simulink model "raibert_hopper_2d"  (R2014b)
settings: Solver=FixedStepDiscrete  StartTime=0.0  StopTime=inf  FixedStep=sample_time  RelTol=1e-3
undefined symbols (not defined in the file): boom_mount_angle, boom_pelvis_offset_angle, contact_threshold, control_start_time, d_y_boom_com_offset, desired_torso_angle, dt_thrust, dx_avg_desired, dx_avg_samples, dx_desired_step, extra_leg_damping, F_thrust, fcut_contact, g, h_boom, HIP_MTR_MAX_CONT_TORQUE, initial_dt, k_placement, k_sea, kd_flight, kd_lateral, kd_leg_angle, kd_leg_length_secondary, kd_torso, kd_virtual, kp_flight_max, kp_flight_min, kp_lateral, kp_leg_angle, kp_leg_length_secondary, kp_torso, kp_virtual, l0_virtual, l_boom_projected, l_max, l_min, l_retract, l_seg, l_yaw_center_to_pelvis, lambda1, lambda2, lateral_offset, lateral_target_angle_left, lateral_target_angle_right, leg_length_secondary, loaded_threshold, m_leg_motor, m_total_real, max_leg_angle, max_torque_lateral, max_torque_sagittal, maximum_lateral_angle, min_leg_angle, minimum_lateral_angle, sample_time, t_flight, x_limit
libraries: simulink x7
(part 1 of 2)
settings Model: xpc_rtwmakecfg_data=_xpcethercatlib_  BufferReuse=off  Creator=wmartin  LastModifiedBy=wmartin
settings SolverCC: EnableConcurrentExecution=on
settings DataIOCC: MaxDataPoints=1000000000  SaveFormat=StructureWithTime
settings OptimizationCC: BlockReduction=off  OptimizeBlockIOStorage=off  BufferReuse=off  GlobalBufferReuse=off  ExpressionFolding=off  ExpressionDepthLimit=2147483647  LocalBlockOutputs=off  SimCompilerOptimization=On
settings DebuggingCC: UnderspecifiedInitializationDetection=Classic  MergeDetectMultiDrivingBlocksExec=none  StateNameClashWarn=warning
settings HardwareCC: ProdIntDivRoundTo=Zero  ProdEndianess=LittleEndian  ProdLongLongMode=on  ProdHWDeviceType=Generic->32-bit x86 compatible
settings ModelReferenceCC: UpdateModelReferenceTargets=IfOutOfDate  EnableParallelModelReferenceBuilds=on
settings RTWCC: SystemTargetFile=slrt.tlc  TemplateMakefile=slrt_default_tmf  Description=Simulink Real-Time  RTWVerbose=off  ProcessScript=slrt_make_rtw_hook  RTWCompilerOptimization=On
settings CodeAppCC: MaxIdLength=256
settings SimulinkRealTimeCC: GeneratePreprocessorConditionals=Disable all  EnableShiftOperators=on  RL32LogBufSizeModifier=100000000

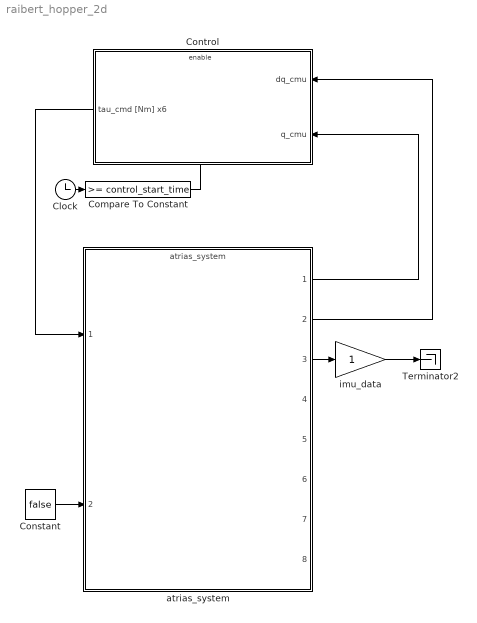
== system raibert_hopper_2d ==
  Clock : Clock
  Compare To Constant : simulink/Logic and Bit Operations/Compare To Constant  relop=>=  const=control_start_time  OutDataTypeStr=boolean
  Constant : Constant  Value=false
  Control : Subsystem
  Terminator2 : Terminator
  atrias_system : ModelReference  ModelNameDialog=atrias_system  SimulationMode=Normal  ModelReferenceVersion=1.2644  CopyOfModelName=atrias_system  DefaultDataLogging=on
  imu_data : Gain
  wires:
  Clock/1 -> Compare To Constant/1
  Compare To Constant/1 -> Control/Enable
  atrias_system/1 -> Control/2(q_cmu)
  atrias_system/2 -> Control/1(dq_cmu)
  Constant/1 -> atrias_system/2
  Control/1(tau_cmd [Nm] x6) -> atrias_system/1
  imu_data/1 -> Terminator2/1
  atrias_system/3 -> imu_data/1

== system raibert_hopper_2d/Control ==
  dq_cmu : Inport
  q_cmu : Inport  Port=2
  Enable : EnablePort  StatesWhenEnabling=reset
  Actuator Control : ModelReference  ModelNameDialog=actuator_control  SimulationMode=Normal  ModelReferenceVersion=1.25  CopyOfModelName=actuator_control  DefaultDataLogging=on
  Behavior Control : Subsystem
  Constant : Constant  Value=[true true true true]  OutDataTypeStr=boolean
  tau_cmd [Nm] x6 : Outport  InitialOutput=[0 0 0 0 0 0]
  wires:
  q_cmu/1 -> Behavior Control/2(q_cmu), Actuator Control/3
  dq_cmu/1 -> Behavior Control/1(dq_cmu), Actuator Control/4
  Behavior Control/1(motor_torque_cmd) -> Actuator Control/1
  Actuator Control/1 -> tau_cmd [Nm] x6/1
  Constant/1 -> Actuator Control/2

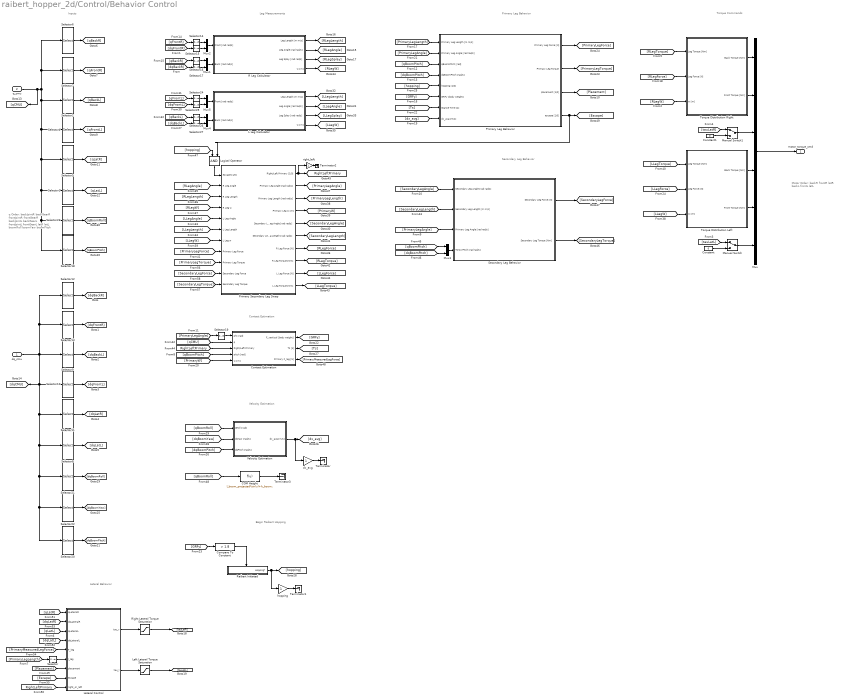
== system raibert_hopper_2d/Control/Behavior Control ==
  note: Begin Raibert Hopping
  note: Velocity Estimation
  note: Contact Estimation
  note: Leg Measurements
  note: Lateral Behavior
  note: Torque Commands
  note: Secondary Leg Behavior
  note: Primary Leg Behavior
  note: Inputs
  note: q Order:
      |
      | backJointR
      | backGearR
      | frontJointR
      | frontGearR
      |
      | backJointL
      | backGearL
      | frontJointL
      | frontGearL
      |
      | latR
      | latL
      |
      | boomRoll
      | boomYaw
      | boomPitch
  note: Motor Order:
      |
      | backR
      | frontR
      | latR
      | backL
      | frontL
      | latL
  dq_cmu : Inport
  q_cmu : Inport  Port=2
  COM Height : Fcn  Expr=l_boom_projected*sin(u)+h_boom;
  Compare To Constant : simulink/Logic and Bit Operations/Compare To Constant  relop=>  const=1.8  OutDataTypeStr=boolean
  Constant : Constant  Value=0
  Constant1 : Constant  Value=0
  Contact Estimation : Subsystem
  L Leg Calculator : Subsystem
  Lateral Control : MATLAB Function  TreatAsAtomicUnit=on
  Left Lateral Torque Saturation : Saturate  UpperLimit=max_torque_lateral  LowerLimit=-max_torque_lateral
      settings: AttributesFormatString=Top: %<UpperLimit>\nBottom: %<LowerLimit>
  Logical Operator : Logic  IconShape=distinctive  AllPortsSameDT=off  OutDataTypeStr=boolean
  Manual Switch : ManualSwitch
  Manual Switch1 : ManualSwitch
  Mux : Mux  Inputs=6
  Mux{1..5} (5 alike) : Mux  Inputs=2
  Primary Leg Behavior : Subsystem
  Primary Secondary Leg Swap : Subsystem
  R Leg Calculator : Subsystem
  Raibert Initiated : Subsystem
  Right Lateral Torque Saturation : Saturate  UpperLimit=max_torque_lateral  LowerLimit=-max_torque_lateral
      settings: AttributesFormatString=Top: %<UpperLimit>\nBottom: %<LowerLimit>
  Secondary Leg Behavior : Subsystem
  Selector{,14..17,19,24..27} (10 alike) : Selector  InputPortWidth=2  Indices=[1]
  Selector1 : Selector  InputPortWidth=13  Indices=[10]
  Selector10 : Selector  InputPortWidth=13  Indices=[7 8]
  Selector11 : Selector  InputPortWidth=13  Indices=[9]
  Selector12 : Selector  InputPortWidth=13  Indices=[1 2]
  Selector13 : Selector  InputPortWidth=13  Indices=[3 4]
  Selector18 : Selector  InputPortWidth=13  Indices=[13]
  Selector2 : Selector  InputPortWidth=13  Indices=[5 6]
  Selector20 : Selector  InputPortWidth=13  Indices=[13]
  Selector21 : Selector  InputPortWidth=13  Indices=[11]
  Selector22 : Selector  InputPortWidth=13  Indices=[12]
  Selector23 : Selector  InputPortWidth=13  Indices=[11]
  Selector4 : Selector  InputPortWidth=13  Indices=[7 8]
  Selector5 : Selector  InputPortWidth=13  Indices=[9]
  Selector6 : Selector  InputPortWidth=13  Indices=[1 2]
  Selector7 : Selector  InputPortWidth=13  Indices=[3 4]
  Selector8 : Selector  InputPortWidth=13  Indices=[10]
  Selector9 : Selector  InputPortWidth=13  Indices=[5 6]
  Terminator{,1..3} (4 alike) : Terminator
  Torque Distribution Left : Subsystem
  Torque Distribution Right : Subsystem
  Velocity Estimation : Subsystem
  dx_avg : Gain
  hopping : Gain
  right_left : Gain
  motor_torque_cmd : Outport  OutputWhenDisabled=reset  InitialOutput=[0 0 0 0 0 0]
  tag scope: RightLeftPrimary=global
  wires:
  Compare To Constant/1 -> Raibert Initiated/Enable
  COM Height/1 -> Terminator3/1
  [qBoomRoll] -> COM Height/1
  Logical Operator/1 -> Primary Secondary Leg Swap/1(escape [1/0])
  [hopping] -> Logical Operator/1
  right_left/1 -> Terminator2/1
  Mux3/1 -> Secondary Leg Behavior/4(Torso Pitch [rad rad/s])
  [dqBoomPitch] -> Mux3/2
  [qBoomPitch] -> Mux3/1
  [SecondaryLegLength] -> Secondary Leg Behavior/2(Secondary Leg Length [m m/s])
  [SecondaryLegAngle] -> Secondary Leg Behavior/1(Secondary Leg Angle [rad rad/s])
  [PrimaryLegAngle] -> Secondary Leg Behavior/3(Primary Leg Angle [rad rad/s])
  Secondary Leg Behavior/2(Secondary Leg Torque [Nm]) -> [SecondaryLegTorque]
  Secondary Leg Behavior/1(Secondary Leg Force [N]) -> [SecondaryLegForce]
  [RightLeftPrimary] -> Contact Estimation/3(Right/Left Primary)
  [qCMU] -> Contact Estimation/2(q)
  [LLegW] -> Torque Distribution Left/3(w [m])
  [LLegForce] -> Torque Distribution Left/2(Leg Force [N])
  [LLegTorque] -> Torque Distribution Left/1(Leg Torque [Nm])
  Torque Distribution Left/2(Front Torque [Nm]) -> Mux/5
  Torque Distribution Left/1(Back Torque [Nm]) -> Mux/4
  hopping/1 -> Terminator1/1
  dx_avg/1 -> Terminator/1
  [dqBoomPitch] -> Velocity Estimation/3(dqPitch [rad/s])
  [dqBoomYaw] -> Velocity Estimation/2(dqYaw [rad/s])
  [qBoomRoll] -> Velocity Estimation/1(qRoll [rad])
  Velocity Estimation/1(dx_avg [m/s]) -> [dx_avg], dx_avg/1
  Primary Leg Behavior/2(Primary Leg Torque) -> [PrimaryLegTorque]
  Primary Leg Behavior/1(Primary Leg Force [N]) -> [PrimaryLegForce]
  [dx_avg] -> Primary Leg Behavior/8(dx_avg [m/s])
  [Ts] -> Primary Leg Behavior/7(Stance Time [s])
  [PrimaryLegAngle] -> Primary Leg Behavior/2(Primary Leg Angle [rad rad/s])
  [dqBoomPitch] -> Primary Leg Behavior/4(dqBoomPitch [rad/s])
  [qBoomPitch] -> Primary Leg Behavior/3(qBoomPitch [rad])
  [GRFy] -> Primary Leg Behavior/6(GRFy [body weight])
  [hopping] -> Primary Leg Behavior/5(hopping [1/0])
  [PrimaryLegLength] -> Primary Leg Behavior/1(Primary Leg Length [m m/s])
  Primary Secondary Leg Swap/1(Right/Left Primary [1/0]) -> [RightLeftPrimary], right_left/1
  Primary Leg Behavior/4(escape [1/0]) -> [Escape], Logical Operator/2
  Primary Secondary Leg Swap/10(L Leg Torque [Nm]) -> [LLegTorque]
  Primary Secondary Leg Swap/9(L Leg Force [N]) -> [LLegForce]
  Primary Secondary Leg Swap/8(R Leg Torque [Nm]) -> [RLegTorque]
  Primary Secondary Leg Swap/7(R Leg Force [N]) -> [RLegForce]
  Primary Secondary Leg Swap/4(Primary Leg w [m]) -> [PrimaryW]
  Primary Secondary Leg Swap/3(Primary Leg Length [rad rad/s]) -> [PrimaryLegLength]
  Primary Secondary Leg Swap/2(Primary Leg Angle [rad rad/s]) -> [PrimaryLegAngle]
  Primary Secondary Leg Swap/6(Secondary Leg Length [rad rad/s]) -> [SecondaryLegLength]
  Primary Secondary Leg Swap/5(Secondary Leg Angle [rad rad/s]) -> [SecondaryLegAngle]
  [SecondaryLegTorque] -> Primary Secondary Leg Swap/11(Secondary Leg Torque)
  [SecondaryLegForce] -> Primary Secondary Leg Swap/10(Secondary Leg Force)
  [PrimaryLegTorque] -> Primary Secondary Leg Swap/9(Primary Leg Torque)
  [PrimaryLegForce] -> Primary Secondary Leg Swap/8(Primary Leg Force)
  [RLegW] -> Primary Secondary Leg Swap/4(R Leg w)
  [RLegLength] -> Primary Secondary Leg Swap/3(R Leg Length)
  [RLegAngle] -> Primary Secondary Leg Swap/2(R Leg Angle)
  [LLegW] -> Primary Secondary Leg Swap/7(L Leg w)
  [LLegLength] -> Primary Secondary Leg Swap/6(L Leg Length)
  [LLegAngle] -> Primary Secondary Leg Swap/5(L Leg Angle)
  L Leg Calculator/4(w [m]) -> [LLegW]
  R Leg Calculator/4(w [m]) -> [RLegW]
  Selector26/1 -> Mux4/1
  Selector27/1 -> Mux4/2
  Selector25/1 -> Mux5/2
  Selector24/1 -> Mux5/1
  L Leg Calculator/3(Leg Splay [rad rad/s]) -> [LLegSplay]
  L Leg Calculator/2(Leg Angle [rad rad/s]) -> [LLegAngle]
  L Leg Calculator/1("Leg Length [m m/s] ") -> [LLegLength]
  Mux4/1 -> L Leg Calculator/2(Back [rad rad/s])
  Mux5/1 -> L Leg Calculator/1(Front [rad rad/s])
  [dqFrontL] -> Selector25/1
  [qFrontL] -> Selector24/1
  [dqBackL] -> Selector27/1
  [qBackL] -> Selector26/1
  Selector23/1 -> [qBoomRoll]
  Selector21/1 -> [dqBoomRoll]
  dq_cmu/1 -> Selector9/1, Selector13/1, Selector12/1, [dqCMU], Selector10/1, Selector11/1, Selector8/1, Selector21/1, Selector22/1, Selector20/1
  Raibert Initiated/1(Hopping?) -> [hopping], hopping/1
  [GRFy] -> Compare To Constant/1
  Contact Estimation/2(Ts [s]) -> [Ts]
  Selector22/1 -> [dqBoomYaw]
  [RLegTorque] -> Torque Distribution Right/1(Leg Torque [Nm])
  [RLegForce] -> Torque Distribution Right/2(Leg Force [N])
  Selector20/1 -> [dqBoomPitch]
  Contact Estimation/1(F_vertical [body weight]) -> [GRFy]
  Selector19/1 -> Contact Estimation/1(phi [rad])
  [PrimaryLegAngle] -> Selector19/1
  [qBoomPitch] -> Contact Estimation/4(pitch [rad])
  Selector18/1 -> [qBoomPitch]
  q_cmu/1 -> [qCMU], Selector1/1, Selector23/1, Selector18/1, Selector5/1, Selector4/1, Selector2/1, Selector7/1, Selector6/1
  [PrimaryW] -> Contact Estimation/5(w [m])
  Selector16/1 -> Mux1/1
  Selector17/1 -> Mux1/2
  Selector15/1 -> Mux2/2
  Selector14/1 -> Mux2/1
  [RLegW] -> Torque Distribution Right/3(w [m])
  [tauLatL] -> Manual Switch/1
  [tauLatR] -> Manual Switch1/1
  Torque Distribution Right/2(Front Torque [Nm]) -> Mux/2
  Torque Distribution Right/1(Back Torque [Nm]) -> Mux/1
  R Leg Calculator/3(Leg Splay [rad rad/s]) -> [RLegSplay]
  R Leg Calculator/2(Leg Angle [rad rad/s]) -> [RLegAngle]
  R Leg Calculator/1("Leg Length [m m/s] ") -> [RLegLength]
  Mux1/1 -> R Leg Calculator/2(Back [rad rad/s])
  Mux2/1 -> R Leg Calculator/1(Front [rad rad/s])
  [dqFrontR] -> Selector15/1
  [qFrontR] -> Selector14/1
  [dqBackR] -> Selector17/1
  [qBackR] -> Selector16/1
  Selector10/1 -> [dqFrontL]
  Selector9/1 -> [dqBackL]
  Selector13/1 -> [dqFrontR]
  Selector12/1 -> [dqBackR]
  Selector11/1 -> [dqLatR]
  Selector8/1 -> [dqLatL]
  Mux/1 -> motor_torque_cmd/1
  Manual Switch1/1 -> Mux/3
  Manual Switch/1 -> Mux/6
  Constant/1 -> Manual Switch/2
  Constant1/1 -> Manual Switch1/2
  Selector5/1 -> [qLatR]
  Selector1/1 -> [qLatL]
  Selector6/1 -> [qBackR]
  Selector7/1 -> [qFrontR]
  Selector2/1 -> [qBackL]
  Selector4/1 -> [qFrontL]
  Primary Leg Behavior/3(placement [1/0]) -> [Placement]
  Lateral Control/1(tau_r) -> Right Lateral Torque Saturation/1
  Lateral Control/2(tau_l) -> Left Lateral Torque Saturation/1
  [Placement] -> Lateral Control/7(placement)
  [RightLeftPrimary] -> Lateral Control/9(right_or_left)
  [qLatR] -> Lateral Control/1(qLateralR)
  [qLatL] -> Lateral Control/3(qLateralL)
  [dqLatL] -> Lateral Control/4(dqLateralL)
  [dqLatR] -> Lateral Control/2(dqLateralR)
  [PrimaryLegLength] -> Selector/1
  [PrimaryMeasuredLegForce] -> Lateral Control/5(F_leg)
  Right Lateral Torque Saturation/1 -> [tauLatR]
  Left Lateral Torque Saturation/1 -> [tauLatL]
  Contact Estimation/3(Primary F_leg [N]) -> [PrimaryMeasuredLegForce]
  Selector/1 -> Lateral Control/6(l_leg)
  [Escape] -> Lateral Control/8(escape)

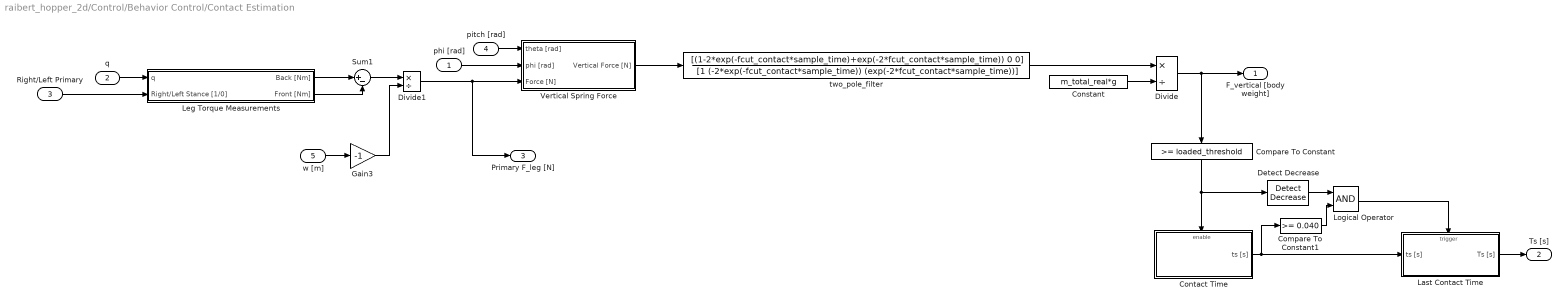
== system raibert_hopper_2d/Control/Behavior Control/Contact Estimation ==
  phi [rad] : Inport
  q : Inport  Port=2
  Right/Left Primary : Inport  Port=3
  pitch [rad] : Inport  Port=4
  w [m] : Inport  Port=5
  Compare To Constant : simulink/Logic and Bit Operations/Compare To Constant  relop=>=  const=loaded_threshold  OutDataTypeStr=boolean
  Compare To Constant1 : simulink/Logic and Bit Operations/Compare To Constant  relop=>=  const=0.040  OutDataTypeStr=boolean
  Constant : Constant  Value=m_total_real*g
  Contact Time : Subsystem
  Detect Decrease : simulink/Logic and Bit Operations/Detect Decrease  vinit=0.0  InputProcessing=Inherited  OutDataTypeStr=boolean
  Divide : Product  Inputs=*/
  Divide1 : Product  Inputs=*/
  Gain3 : Gain  Gain=-1
  Last Contact Time : Subsystem
  Leg Torque Measurements : Subsystem
  Logical Operator : Logic  AllPortsSameDT=off  OutDataTypeStr=boolean
  Sum1 : Sum  Inputs=|+-
  Vertical Spring Force : Subsystem
  two_pole_filter : DiscreteTransferFcn  Numerator=[(1-2*exp(-fcut_contact*sample_time)+exp(-2*fcut_contact*sample_time)) 0 0]  Denominator=[1 (-2*exp(-fcut_contact*sample_time)) (exp(-2*fcut_contact*sample_time))]  SampleTime=sample_time
  F_vertical [body weight] : Outport
  Ts [s] : Outport  Port=2
  Primary F_leg [N] : Outport  Port=3
  wires:
  Right/Left Primary/1 -> Leg Torque Measurements/2(Right/Left Stance [1/0])
  Compare To Constant1/1 -> Logical Operator/2
  Detect Decrease/1 -> Logical Operator/1
  Logical Operator/1 -> Last Contact Time/Trigger
  Divide/1 -> Compare To Constant/1, F_vertical [body weight]/1
  Compare To Constant/1 -> Contact Time/Enable, Detect Decrease/1
  Contact Time/1(ts [s]) -> Compare To Constant1/1, Last Contact Time/1(ts [s])
  Last Contact Time/1(Ts [s]) -> Ts [s]/1
  phi [rad]/1 -> Vertical Spring Force/2(phi [rad])
  Gain3/1 -> Divide1/2
  w [m]/1 -> Gain3/1
  pitch [rad]/1 -> Vertical Spring Force/1(theta [rad])
  Divide1/1 -> Primary F_leg [N]/1, Vertical Spring Force/3(Force [N])
  Sum1/1 -> Divide1/1
  Leg Torque Measurements/2(Front [Nm]) -> Sum1/2
  Leg Torque Measurements/1(Back [Nm]) -> Sum1/1
  q/1 -> Leg Torque Measurements/1(q)
  two_pole_filter/1 -> Divide/1
  Constant/1 -> Divide/2
  Vertical Spring Force/1(Vertical Force [N]) -> two_pole_filter/1

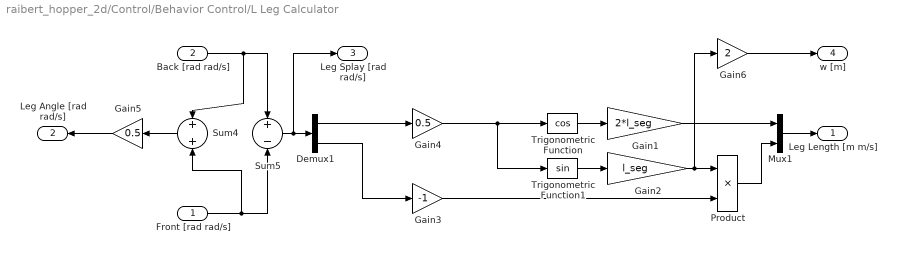
== system raibert_hopper_2d/Control/Behavior Control/L Leg Calculator ==
  Front [rad rad/s] : Inport
  Back [rad rad/s] : Inport  Port=2
  Demux1 : Demux  Outputs=2
  Gain1 : Gain  Gain=2*l_seg
  Gain2 : Gain  Gain=l_seg
  Gain3 : Gain  Gain=-1
  Gain4 : Gain  Gain=0.5
  Gain5 : Gain  Gain=0.5
  Gain6 : Gain  Gain=2
  Mux1 : Mux  Inputs=2
  Product : Product  RndMeth=Zero
  Sum4 : Sum  Inputs=+|+
  Sum5 : Sum  Inputs=+|-
  Trigonometric Function : Trigonometry  Operator=cos
  Trigonometric Function1 : Trigonometry
  "Leg Length [m m/s] " : Outport
  Leg Angle [rad rad/s] : Outport  Port=2
  Leg Splay [rad rad/s] : Outport  Port=3
  w [m] : Outport  Port=4
  wires:
  Gain6/1 -> w [m]/1
  Gain4/1 -> Trigonometric Function1/1, Trigonometric Function/1
  Trigonometric Function/1 -> Gain1/1
  Gain1/1 -> Mux1/1
  Trigonometric Function1/1 -> Gain2/1
  Product/1 -> Mux1/2
  Front [rad rad/s]/1 -> Sum5/2, Sum4/2
  Back [rad rad/s]/1 -> Sum4/1, Sum5/1
  Demux1/2 -> Gain3/1
  Gain3/1 -> Product/2
  Demux1/1 -> Gain4/1
  Gain2/1 -> Product/1, Gain6/1
  Sum5/1 -> Leg Splay [rad rad/s]/1, Demux1/1
  Mux1/1 -> "Leg Length [m m/s] "/1
  Sum4/1 -> Gain5/1
  Gain5/1 -> Leg Angle [rad rad/s]/1

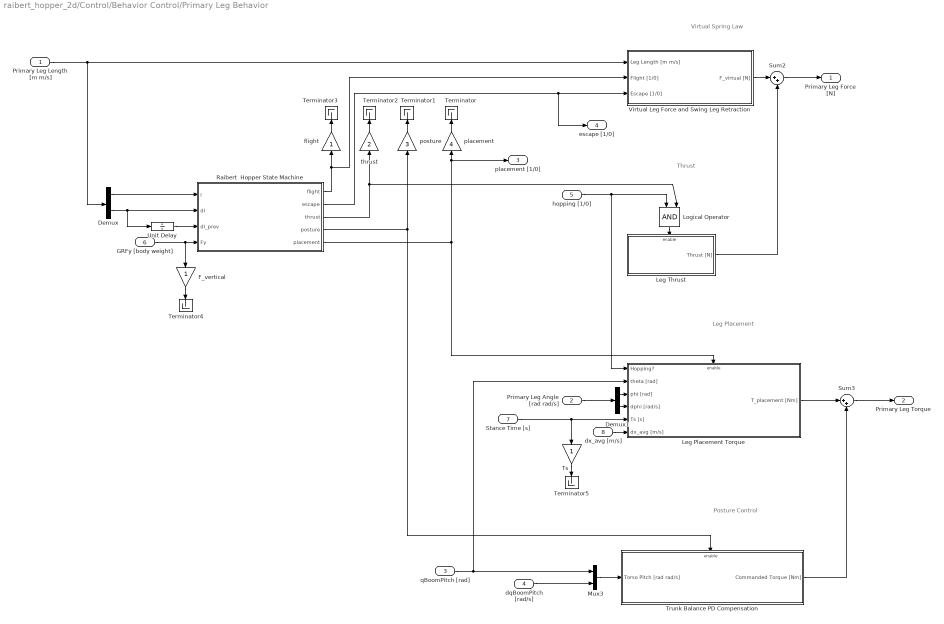
== system raibert_hopper_2d/Control/Behavior Control/Primary Leg Behavior ==
  note: Leg Placement
  note: Posture Control
  note: Thrust
  note: Virtual Spring Law
  Primary Leg Length [m m/s] : Inport
  Primary Leg Angle [rad rad/s] : Inport  Port=2
  qBoomPitch [rad] : Inport  Port=3
  dqBoomPitch [rad/s] : Inport  Port=4
  hopping [1/0] : Inport  Port=5
  GRFy [body weight] : Inport  Port=6
  Stance Time [s] : Inport  Port=7
  dx_avg [m/s] : Inport  Port=8
  Demux : Demux  Outputs=2
  Demux1 : Demux  Outputs=2
  F_vertical : Gain
  Leg Placement Torque : Subsystem
  Leg Thrust : Subsystem
  Logical Operator : Logic  IconShape=distinctive  AllPortsSameDT=off  OutDataTypeStr=boolean
  Mux3 : Mux  Inputs=2
  Raibert  Hopper State Machine : State Transition Table  TreatAsAtomicUnit=on
  Sum2 : Sum  Inputs=|++
  Sum3 : Sum  Inputs=|++
  Terminator{,1..5} (6 alike) : Terminator
  Trunk Balance PD Compensation : Subsystem
  Ts : Gain
  Unit Delay : UnitDelay  SampleTime=-1
  Virtual Leg Force and Swing Leg Retraction : Subsystem
  flight : Gain
  placement : Gain  Gain=4
  posture : Gain  Gain=3
  thrust : Gain  Gain=2
  Primary Leg Force [N] : Outport
  Primary Leg Torque : Outport  Port=2
  placement [1/0] : Outport  Port=3  OutDataTypeStr=boolean
  escape [1/0] : Outport  Port=4
  wires:
  hopping [1/0]/1 -> Logical Operator/1, Leg Placement Torque/1(Hopping?)
  Ts/1 -> Terminator5/1
  Demux/1 -> Raibert  Hopper State Machine/1(l)
  flight/1 -> Terminator3/1
  F_vertical/1 -> Terminator4/1
  Primary Leg Length [m m/s]/1 -> Virtual Leg Force and Swing Leg Retraction/1(Leg Length [m m/s]), Demux/1
  thrust/1 -> Terminator2/1
  posture/1 -> Terminator1/1
  Logical Operator/1 -> Leg Thrust/Enable
  Raibert  Hopper State Machine/5(placement) -> placement [1/0]/1, placement/1, Leg Placement Torque/Enable
  Stance Time [s]/1 -> Ts/1, Leg Placement Torque/5(Ts [s])
  Primary Leg Angle [rad rad/s]/1 -> Demux1/1
  Demux1/2 -> Leg Placement Torque/4(dphi [rad/s])
  Demux1/1 -> Leg Placement Torque/3(phi [rad])
  dx_avg [m/s]/1 -> Leg Placement Torque/6(dx_avg [m/s])
  Sum3/1 -> Primary Leg Torque/1
  Leg Placement Torque/1(T_placement [Nm]) -> Sum3/1
  Raibert  Hopper State Machine/2(escape) -> Virtual Leg Force and Swing Leg Retraction/3(Escape [1/0]), escape [1/0]/1
  Virtual Leg Force and Swing Leg Retraction/1(F_virtual [N]) -> Sum2/1
  Raibert  Hopper State Machine/1(flight) -> Virtual Leg Force and Swing Leg Retraction/2(Flight [1/0]), flight/1
  Sum2/1 -> Primary Leg Force [N]/1
  Leg Thrust/1(Thrust [N]) -> Sum2/2
  Raibert  Hopper State Machine/3(thrust) -> thrust/1, Logical Operator/2
  Demux/2 -> Raibert  Hopper State Machine/2(dl), Unit Delay/1
  GRFy [body weight]/1 -> Raibert  Hopper State Machine/4(Fy), F_vertical/1
  Unit Delay/1 -> Raibert  Hopper State Machine/3(dl_prev)
  Trunk Balance PD Compensation/1(Commanded Torque [Nm]) -> Sum3/2
  dqBoomPitch [rad/s]/1 -> Mux3/2
  qBoomPitch [rad]/1 -> Leg Placement Torque/2(theta [rad]), Mux3/1
  Mux3/1 -> Trunk Balance PD Compensation/1(Torso Pitch [rad rad/s])
  Raibert  Hopper State Machine/4(posture) -> posture/1, Trunk Balance PD Compensation/Enable
  placement/1 -> Terminator/1

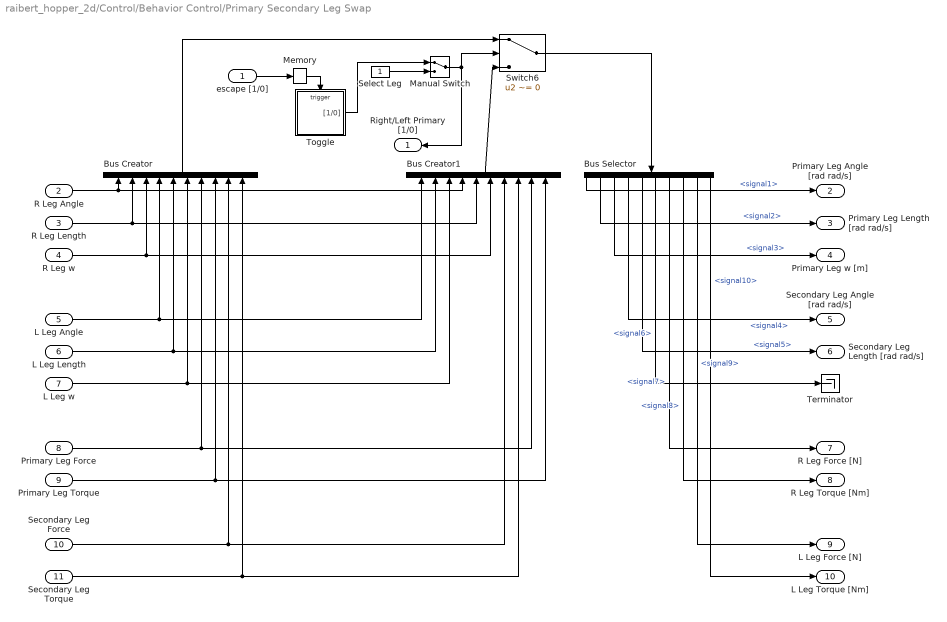
== system raibert_hopper_2d/Control/Behavior Control/Primary Secondary Leg Swap ==
  escape [1/0] : Inport
  R Leg Angle : Inport  Port=2
  R Leg Length : Inport  Port=3
  R Leg w : Inport  Port=4
  L Leg Angle : Inport  Port=5
  L Leg Length : Inport  Port=6
  L Leg w : Inport  Port=7
  Primary Leg Force : Inport  Port=8
  Primary Leg Torque : Inport  Port=9
  Secondary Leg Force : Inport  Port=10
  Secondary Leg Torque : Inport  Port=11
  Bus Creator : BusCreator  Inputs=10
  Bus Creator1 : BusCreator  Inputs=10
  Bus Selector : BusSelector  OutputSignals=signal1,signal2,signal3,signal4,signal5,signal6,signal7,signal8,signal9,signal10
  Manual Switch : ManualSwitch
  Memory : Memory  InheritSampleTime=on
  Select Leg : Constant  OutDataTypeStr=boolean
  Switch6 : Switch  Criteria=u2 ~= 0  ZeroCross=off
  Terminator : Terminator
  Toggle : Subsystem
  Right/Left Primary [1/0] : Outport
  Primary Leg Angle [rad rad/s] : Outport  Port=2
  Primary Leg Length [rad rad/s] : Outport  Port=3
  Primary Leg w [m] : Outport  Port=4
  Secondary Leg Angle [rad rad/s] : Outport  Port=5
  Secondary Leg Length [rad rad/s] : Outport  Port=6
  R Leg Force [N] : Outport  Port=7
  R Leg Torque [Nm] : Outport  Port=8
  L Leg Force [N] : Outport  Port=9
  L Leg Torque [Nm] : Outport  Port=10
  wires:
  Memory/1 -> Toggle/Trigger
  Toggle/1("[1/0]") -> Manual Switch/1
  Manual Switch/1 -> Right/Left Primary [1/0]/1, Switch6/2
  Select Leg/1 -> Manual Switch/2
  Bus Selector/10 -> L Leg Torque [Nm]/1  "<signal10>"
  Bus Selector/9 -> L Leg Force [N]/1  "<signal9>"
  Bus Selector/8 -> R Leg Torque [Nm]/1  "<signal8>"
  Bus Selector/7 -> R Leg Force [N]/1  "<signal7>"
  Bus Selector/6 -> Terminator/1  "<signal6>"
  Bus Selector/5 -> Secondary Leg Length [rad rad/s]/1  "<signal5>"
  Bus Selector/4 -> Secondary Leg Angle [rad rad/s]/1  "<signal4>"
  Bus Selector/3 -> Primary Leg w [m]/1  "<signal3>"
  Bus Selector/2 -> Primary Leg Length [rad rad/s]/1  "<signal2>"
  Bus Selector/1 -> Primary Leg Angle [rad rad/s]/1  "<signal1>"
  L Leg Angle/1 -> Bus Creator1/1, Bus Creator/4
  L Leg Length/1 -> Bus Creator1/2, Bus Creator/5
  Primary Leg Force/1 -> Bus Creator/7, Bus Creator1/9
  R Leg w/1 -> Bus Creator/3, Bus Creator1/6
  R Leg Angle/1 -> Bus Creator/1, Bus Creator1/4
  L Leg w/1 -> Bus Creator1/3, Bus Creator/6
  R Leg Length/1 -> Bus Creator/2, Bus Creator1/5
  escape [1/0]/1 -> Memory/1
  Secondary Leg Force/1 -> Bus Creator/9, Bus Creator1/7
  Secondary Leg Torque/1 -> Bus Creator/10, Bus Creator1/8
  Primary Leg Torque/1 -> Bus Creator/8, Bus Creator1/10
  Bus Creator/1 -> Switch6/1
  Bus Creator1/1 -> Switch6/3
  Switch6/1 -> Bus Selector/1

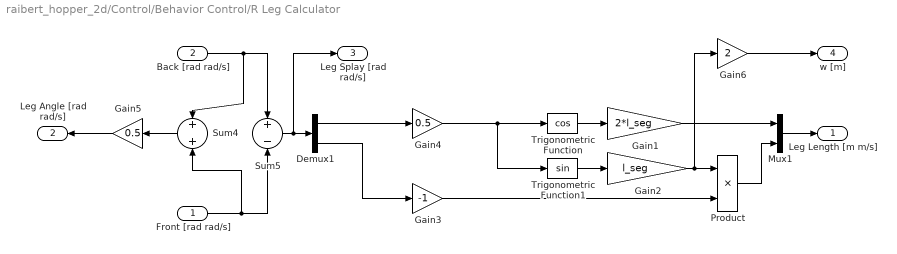
== system raibert_hopper_2d/Control/Behavior Control/R Leg Calculator ==
  Front [rad rad/s] : Inport
  Back [rad rad/s] : Inport  Port=2
  Demux1 : Demux  Outputs=2
  Gain1 : Gain  Gain=2*l_seg
  Gain2 : Gain  Gain=l_seg
  Gain3 : Gain  Gain=-1
  Gain4 : Gain  Gain=0.5
  Gain5 : Gain  Gain=0.5
  Gain6 : Gain  Gain=2
  Mux1 : Mux  Inputs=2
  Product : Product  RndMeth=Zero
  Sum4 : Sum  Inputs=+|+
  Sum5 : Sum  Inputs=+|-
  Trigonometric Function : Trigonometry  Operator=cos
  Trigonometric Function1 : Trigonometry
  "Leg Length [m m/s] " : Outport
  Leg Angle [rad rad/s] : Outport  Port=2
  Leg Splay [rad rad/s] : Outport  Port=3
  w [m] : Outport  Port=4
  wires:
  Gain5/1 -> Leg Angle [rad rad/s]/1
  Sum4/1 -> Gain5/1
  Mux1/1 -> "Leg Length [m m/s] "/1
  Sum5/1 -> Demux1/1, Leg Splay [rad rad/s]/1
  Gain2/1 -> Gain6/1, Product/1
  Demux1/1 -> Gain4/1
  Gain3/1 -> Product/2
  Demux1/2 -> Gain3/1
  Back [rad rad/s]/1 -> Sum5/1, Sum4/1
  Front [rad rad/s]/1 -> Sum4/2, Sum5/2
  Product/1 -> Mux1/2
  Trigonometric Function1/1 -> Gain2/1
  Gain1/1 -> Mux1/1
  Trigonometric Function/1 -> Gain1/1
  Gain4/1 -> Trigonometric Function/1, Trigonometric Function1/1
  Gain6/1 -> w [m]/1

== system raibert_hopper_2d/Control/Behavior Control/Raibert Initiated ==
  Enable : EnablePort  StatesWhenEnabling=reset
  Constant : Constant
  Hopping? : Outport  InitialOutput=[0]
  wires:
  Constant/1 -> Hopping?/1

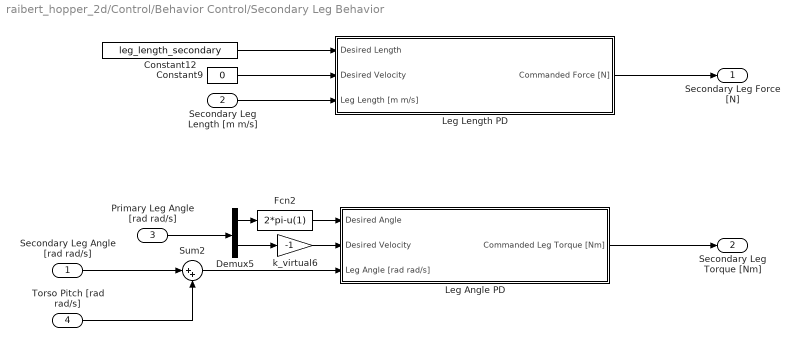
== system raibert_hopper_2d/Control/Behavior Control/Secondary Leg Behavior ==
  Secondary Leg Angle [rad rad/s] : Inport
  Secondary Leg Length [m m/s] : Inport  Port=2
  Primary Leg Angle [rad rad/s] : Inport  Port=3
  Torso Pitch [rad rad/s] : Inport  Port=4
  Constant12 : Constant  Value=leg_length_secondary
  Constant9 : Constant  Value=0
  Demux5 : Demux  Outputs=2
  Fcn2 : Fcn  Expr=2*pi-u(1)
  Leg Angle PD : Subsystem
  Leg Length PD : Subsystem
  Sum2 : Sum  Inputs=|++
  k_virtual6 : Gain  Gain=-1
  Secondary Leg Force [N] : Outport
  Secondary Leg Torque [Nm] : Outport  Port=2
  wires:
  Leg Angle PD/1(Commanded Leg Torque [Nm]) -> Secondary Leg Torque [Nm]/1
  Demux5/2 -> k_virtual6/1
  Demux5/1 -> Fcn2/1
  Primary Leg Angle [rad rad/s]/1 -> Demux5/1
  k_virtual6/1 -> Leg Angle PD/2(Desired Velocity)
  Fcn2/1 -> Leg Angle PD/1(Desired Angle)
  Sum2/1 -> Leg Angle PD/3(Leg Angle [rad rad/s])
  Torso Pitch [rad rad/s]/1 -> Sum2/2
  Secondary Leg Angle [rad rad/s]/1 -> Sum2/1
  Leg Length PD/1(Commanded Force [N]) -> Secondary Leg Force [N]/1
  Secondary Leg Length [m m/s]/1 -> Leg Length PD/3(Leg Length [m m/s])
  Constant12/1 -> Leg Length PD/1(Desired Length)
  Constant9/1 -> Leg Length PD/2(Desired Velocity)

== system raibert_hopper_2d/Control/Behavior Control/Torque Distribution Left ==
  Leg Torque [Nm] : Inport
  Leg Force [N] : Inport  Port=2
  w [m] : Inport  Port=3
  Gain : Gain  Gain=0.5
  Gain1 : Gain  Gain=0.5
  Motor Torque Saturation Optimization : MATLAB Function  TreatAsAtomicUnit=on
  Product : Product  RndMeth=Zero
  Sum : Sum  Inputs=|++
  Sum1 : Sum  Inputs=+-|
  Back Torque [Nm] : Outport
  Front Torque [Nm] : Outport  Port=2
  wires:
  Sum1/1 -> Back Torque [Nm]/1
  Leg Torque [Nm]/1 -> Gain/1
  Sum/1 -> Front Torque [Nm]/1
  Motor Torque Saturation Optimization/1(t1) -> Sum/1, Sum1/1
  w [m]/1 -> Product/2
  Motor Torque Saturation Optimization/2(t2) -> Sum1/2, Sum/2
  Leg Force [N]/1 -> Product/1
  Product/1 -> Gain1/1
  Gain1/1 -> Motor Torque Saturation Optimization/2(x2s)
  Gain/1 -> Motor Torque Saturation Optimization/1(x1s)

== system raibert_hopper_2d/Control/Behavior Control/Torque Distribution Right ==
  Leg Torque [Nm] : Inport
  Leg Force [N] : Inport  Port=2
  w [m] : Inport  Port=3
  Gain : Gain  Gain=0.5
  Gain1 : Gain  Gain=0.5
  Motor Torque Saturation Optimization : MATLAB Function  TreatAsAtomicUnit=on
  Product : Product  RndMeth=Zero
  Sum : Sum  Inputs=|++
  Sum1 : Sum  Inputs=+-|
  Back Torque [Nm] : Outport
  Front Torque [Nm] : Outport  Port=2
  wires:
  Gain/1 -> Motor Torque Saturation Optimization/1(x1s)
  Gain1/1 -> Motor Torque Saturation Optimization/2(x2s)
  Product/1 -> Gain1/1
  Leg Force [N]/1 -> Product/1
  Motor Torque Saturation Optimization/2(t2) -> Sum/2, Sum1/2
  w [m]/1 -> Product/2
  Motor Torque Saturation Optimization/1(t1) -> Sum1/1, Sum/1
  Sum/1 -> Front Torque [Nm]/1
  Leg Torque [Nm]/1 -> Gain/1
  Sum1/1 -> Back Torque [Nm]/1

== system raibert_hopper_2d/Control/Behavior Control/Velocity Estimation ==
  qRoll [rad] : Inport
  dqYaw [rad/s] : Inport  Port=2
  dqPitch [rad/s] : Inport  Port=3
  Recursive Moving Average : Subsystem
  dx_from_yaw_and_roll : MATLAB Function  TreatAsAtomicUnit=on
  dx_avg [m/s] : Outport
  wires:
  dqPitch [rad/s]/1 -> dx_from_yaw_and_roll/3(dqPitch)
  qRoll [rad]/1 -> dx_from_yaw_and_roll/1(qRoll)
  dqYaw [rad/s]/1 -> dx_from_yaw_and_roll/2(dqYaw)
  dx_from_yaw_and_roll/1(dx) -> Recursive Moving Average/1(dx [m/s])
  Recursive Moving Average/1(dx_avg [m/s]) -> dx_avg [m/s]/1

== system raibert_hopper_2d/Control/Behavior Control/Contact Estimation/Contact Time ==
  Enable : EnablePort  StatesWhenEnabling=reset  ShowOutputPort=on
  Constant : Constant
  Discrete-Time Integrator : DiscreteIntegrator  IntegratorMethod=Accumulation: Forward Euler  gainval=sample_time  ExternalReset=rising  SampleTime=sample_time
  ts [s] : Outport  InitialOutput=[0]
  wires:
  Discrete-Time Integrator/1 -> ts [s]/1
  Enable/1 -> Discrete-Time Integrator/2
  Constant/1 -> Discrete-Time Integrator/1

== system raibert_hopper_2d/Control/Behavior Control/Contact Estimation/Last Contact Time ==
  ts [s] : Inport
  Trigger : TriggerPort  TriggerType=falling  PortDimensions=1
  Ts [s] : Outport  InitialOutput=[initial_dt]
  wires:
  ts [s]/1 -> Ts [s]/1

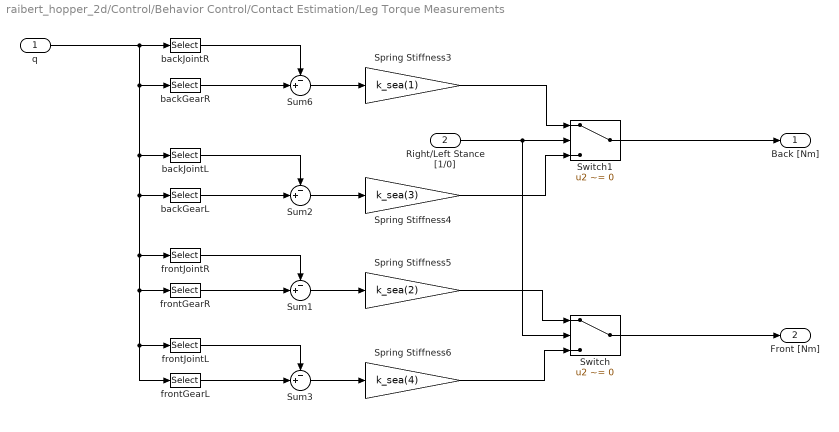
== system raibert_hopper_2d/Control/Behavior Control/Contact Estimation/Leg Torque Measurements ==
  q : Inport
  Right/Left Stance [1/0] : Inport  Port=2
  Spring Stiffness3 : Gain  Gain=k_sea(1)
  Spring Stiffness4 : Gain  Gain=k_sea(3)
  Spring Stiffness5 : Gain  Gain=k_sea(2)
  Spring Stiffness6 : Gain  Gain=k_sea(4)
  Sum{1..3,6} (4 alike) : Sum  Inputs=-+|
  Switch : Switch  Criteria=u2 ~= 0
  Switch1 : Switch  Criteria=u2 ~= 0
  backGearL : Selector  InputPortWidth=13  Indices=[6]
  backGearR : Selector  InputPortWidth=13  Indices=[2]
  backJointL : Selector  InputPortWidth=13  Indices=[5]
  backJointR : Selector  InputPortWidth=13  Indices=[1]
  frontGearL : Selector  InputPortWidth=13  Indices=[8]
  frontGearR : Selector  InputPortWidth=13  Indices=[4]
  frontJointL : Selector  InputPortWidth=13  Indices=[7]
  frontJointR : Selector  InputPortWidth=13  Indices=[3]
  Back [Nm] : Outport
  Front [Nm] : Outport  Port=2
  wires:
  Spring Stiffness6/1 -> Switch/3
  Spring Stiffness5/1 -> Switch/1
  Spring Stiffness4/1 -> Switch1/3
  Spring Stiffness3/1 -> Switch1/1
  q/1 -> backJointR/1, frontGearL/1, frontJointL/1, frontGearR/1, frontJointR/1, backGearL/1, backJointL/1, backGearR/1
  backGearR/1 -> Sum6/2
  frontJointR/1 -> Sum1/1
  frontGearR/1 -> Sum1/2
  backJointR/1 -> Sum6/1
  Switch/1 -> Front [Nm]/1
  Sum1/1 -> Spring Stiffness5/1
  Sum6/1 -> Spring Stiffness3/1
  backGearL/1 -> Sum2/2
  frontJointL/1 -> Sum3/1
  frontGearL/1 -> Sum3/2
  backJointL/1 -> Sum2/1
  Switch1/1 -> Back [Nm]/1
  Sum2/1 -> Spring Stiffness4/1
  Sum3/1 -> Spring Stiffness6/1
  Right/Left Stance [1/0]/1 -> Switch/2, Switch1/2

== system raibert_hopper_2d/Control/Behavior Control/Contact Estimation/Vertical Spring Force ==
  theta [rad] : Inport
  phi [rad] : Inport  Port=2
  Force [N] : Inport  Port=3
  Gain : Gain  Gain=-1
  Product : Product
  Sum : Sum  Inputs=++|
  Trigonometric Function : Trigonometry  Operator=cos
  Vertical Force [N] : Outport
  wires:
  Gain/1 -> Vertical Force [N]/1
  Sum/1 -> Trigonometric Function/1
  Product/1 -> Gain/1
  Trigonometric Function/1 -> Product/2
  theta [rad]/1 -> Sum/1
  phi [rad]/1 -> Sum/2
  Force [N]/1 -> Product/1

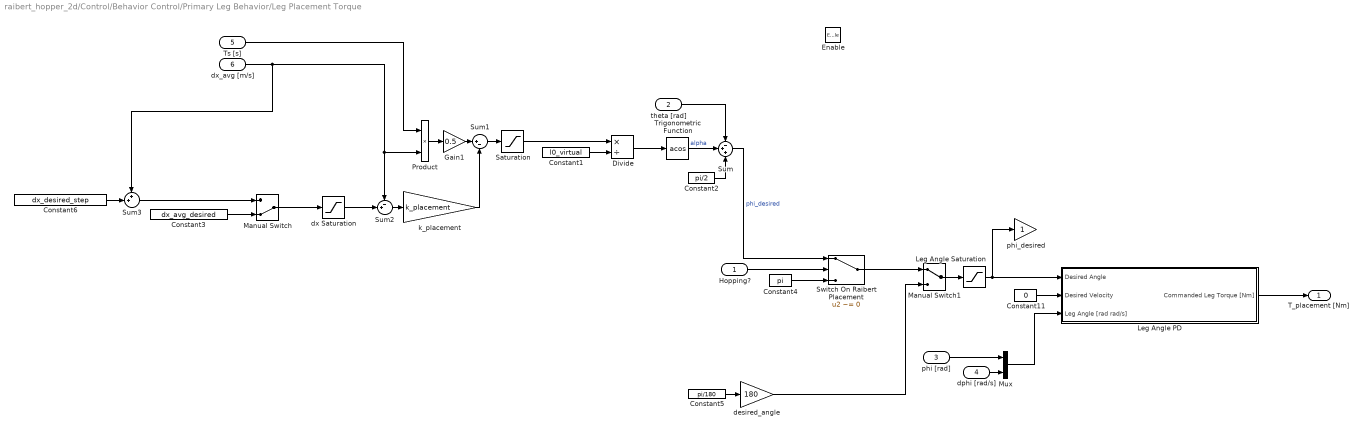
== system raibert_hopper_2d/Control/Behavior Control/Primary Leg Behavior/Leg Placement Torque ==
  Hopping? : Inport
  theta [rad] : Inport  Port=2
  phi [rad] : Inport  Port=3
  dphi [rad/s] : Inport  Port=4
  Ts [s] : Inport  Port=5
  dx_avg [m/s] : Inport  Port=6
  Enable : EnablePort  StatesWhenEnabling=reset
  Constant1 : Constant  Value=l0_virtual
  Constant11 : Constant  Value=0
  Constant2 : Constant  Value=pi/2
  Constant3 : Constant  Value=dx_avg_desired
  Constant4 : Constant  Value=pi
  Constant5 : Constant  Value=pi/180
  Constant6 : Constant  Value=dx_desired_step
  Divide : Product  Inputs=*/
  Gain1 : Gain  Gain=0.5
  Leg Angle PD : Subsystem
  Leg Angle Saturation : Saturate  UpperLimit=max_leg_angle  LowerLimit=min_leg_angle
      settings: AttributesFormatString=Hi: %<UpperLimit>\nLo: %<LowerLimit>
  Manual Switch : ManualSwitch  CurrentSetting=0
  Manual Switch1 : ManualSwitch
  Mux : Mux  Inputs=2
  Product : Product
  Saturation : Saturate  UpperLimit=x_limit  LowerLimit=-x_limit
      settings: AttributesFormatString=Hi: %<UpperLimit>\nLo: %<LowerLimit>
  Sum : Sum  Inputs=-++
  Sum1 : Sum  Inputs=|+-
  Sum2 : Sum  Inputs=-+|
  Sum3 : Sum  Inputs=++|
  Switch On Raibert Placement : Switch  Criteria=u2 ~= 0
  Trigonometric Function : Trigonometry  Operator=acos
  desired_angle : Gain  Gain=180
  dx Saturation : Saturate  UpperLimit=dx_avg_desired  LowerLimit=0
      settings: AttributesFormatString=Hi: %<UpperLimit>\nLo: %<LowerLimit>
  k_placement : Gain  Gain=k_placement
  phi_desired : Gain
  T_placement [Nm] : Outport  OutputWhenDisabled=reset  InitialOutput=[0]
  wires:
  Manual Switch1/1 -> Leg Angle Saturation/1
  desired_angle/1 -> Manual Switch1/2
  Switch On Raibert Placement/1 -> Manual Switch1/1
  Divide/1 -> Trigonometric Function/1
  Sum3/1 -> Manual Switch/1
  Constant6/1 -> Sum3/2
  dx_avg [m/s]/1 -> Product/2, Sum2/1, Sum3/1
  Constant3/1 -> Manual Switch/2
  Manual Switch/1 -> dx Saturation/1
  Constant5/1 -> desired_angle/1
  Leg Angle Saturation/1 -> Leg Angle PD/1(Desired Angle), phi_desired/1
  Hopping?/1 -> Switch On Raibert Placement/2
  Constant4/1 -> Switch On Raibert Placement/3
  dx Saturation/1 -> Sum2/2
  Sum2/1 -> k_placement/1
  k_placement/1 -> Sum1/2
  Sum1/1 -> Saturation/1
  Sum/1 -> Switch On Raibert Placement/1  "phi_desired"
  theta [rad]/1 -> Sum/1
  Constant2/1 -> Sum/3
  Trigonometric Function/1 -> Sum/2  "alpha"
  Constant1/1 -> Divide/2
  Saturation/1 -> Divide/1
  Gain1/1 -> Sum1/1
  Product/1 -> Gain1/1
  Ts [s]/1 -> Product/1
  dphi [rad/s]/1 -> Mux/2
  phi [rad]/1 -> Mux/1
  Leg Angle PD/1(Commanded Leg Torque [Nm]) -> T_placement [Nm]/1
  Mux/1 -> Leg Angle PD/3(Leg Angle [rad rad/s])
  Constant11/1 -> Leg Angle PD/2(Desired Velocity)

== system raibert_hopper_2d/Control/Behavior Control/Primary Leg Behavior/Leg Thrust ==
  Enable : EnablePort  StatesWhenEnabling=reset  ShowOutputPort=on
  F_thrust : Gain  Gain=F_thrust
  Thrust Timer : Subsystem
  thrust period? : simulink/Logic and Bit Operations/Compare To Constant  relop=<=  const=dt_thrust  OutDataTypeStr=uint8
  Thrust [N] : Outport  OutputWhenDisabled=reset  InitialOutput=[0]
  wires:
  thrust period?/1 -> F_thrust/1
  Enable/1 -> Thrust Timer/Enable
  Thrust Timer/1(timer [s]) -> thrust period?/1
  F_thrust/1 -> Thrust [N]/1

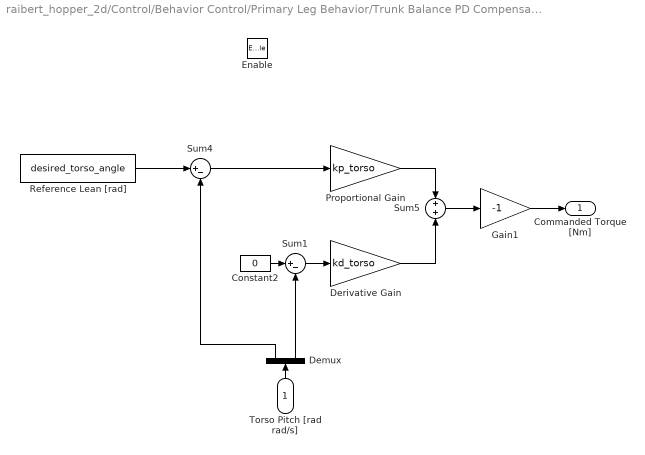
== system raibert_hopper_2d/Control/Behavior Control/Primary Leg Behavior/Trunk Balance PD Compensation ==
  Torso Pitch [rad rad/s] : Inport
  Enable : EnablePort  StatesWhenEnabling=reset
  Constant2 : Constant  Value=0
  Demux : Demux  Outputs=2
  Derivative Gain : Gain  Gain=kd_torso
  Gain1 : Gain  Gain=-1
  Proportional Gain : Gain  Gain=kp_torso
  Reference Lean [rad] : Constant  Value=desired_torso_angle
  Sum1 : Sum  Inputs=|+-
  Sum4 : Sum  Inputs=|+-
  Sum5 : Sum
  Commanded Torque [Nm] : Outport  OutputWhenDisabled=reset  InitialOutput=[0]
  wires:
  Sum5/1 -> Gain1/1
  Demux/2 -> Sum1/2
  Constant2/1 -> Sum1/1
  Reference Lean [rad]/1 -> Sum4/1
  Demux/1 -> Sum4/2
  Sum4/1 -> Proportional Gain/1
  Torso Pitch [rad rad/s]/1 -> Demux/1
  Derivative Gain/1 -> Sum5/2
  Proportional Gain/1 -> Sum5/1
  Sum1/1 -> Derivative Gain/1
  Gain1/1 -> Commanded Torque [Nm]/1

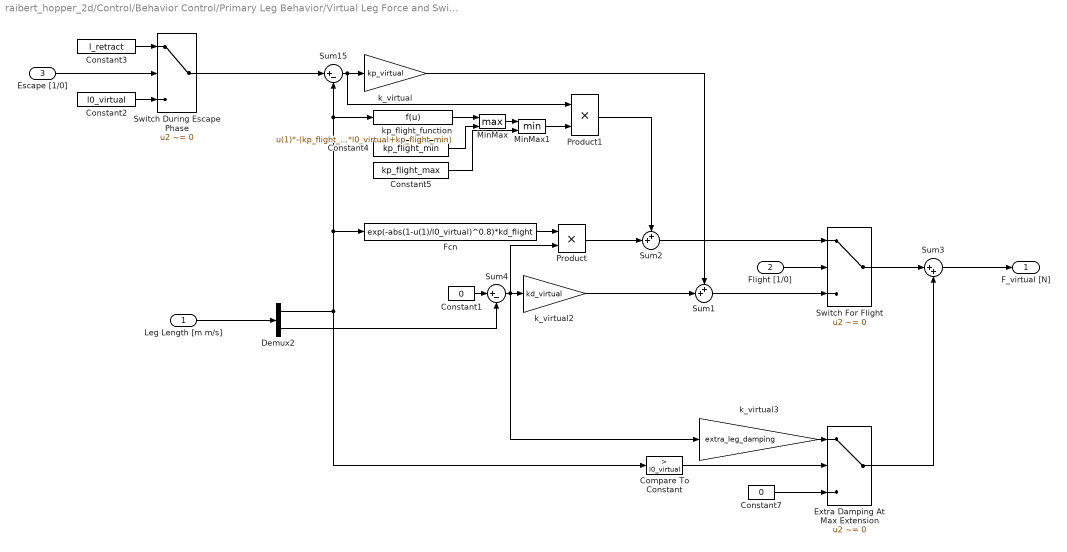
== system raibert_hopper_2d/Control/Behavior Control/Primary Leg Behavior/Virtual Leg Force and Swing Leg Retraction ==
  Leg Length [m m/s] : Inport
  Flight [1/0] : Inport  Port=2
  Escape [1/0] : Inport  Port=3
  Compare To Constant : simulink/Logic and Bit Operations/Compare To Constant  relop=>  const=l0_virtual  OutDataTypeStr=boolean
  Constant1 : Constant  Value=0
  Constant2 : Constant  Value=l0_virtual
  Constant3 : Constant  Value=l_retract
  Constant4 : Constant  Value=kp_flight_min
  Constant5 : Constant  Value=kp_flight_max
  Constant7 : Constant  Value=0
  Demux2 : Demux  Outputs=2
  Extra Damping At Max Extension : Switch  Criteria=u2 ~= 0
  Fcn : Fcn  Expr=exp(-abs(1-u(1)/l0_virtual)^0.8)*kd_flight
  MinMax : MinMax  Function=max  Inputs=2
  MinMax1 : MinMax  Inputs=2
  Product : Product
  Product1 : Product
  Sum1 : Sum  Inputs=++|
  Sum15 : Sum  Inputs=|+-
  Sum2 : Sum  Inputs=++|
  Sum3 : Sum  Inputs=|++
  Sum4 : Sum  Inputs=|+-
  Switch During Escape Phase : Switch  Criteria=u2 ~= 0
  Switch For Flight : Switch  Criteria=u2 ~= 0
  k_virtual : Gain  Gain=kp_virtual
  k_virtual2 : Gain  Gain=kd_virtual
  k_virtual3 : Gain  Gain=extra_leg_damping
  kp_flight_function : Fcn  Expr=u(1)*-(kp_flight_max - kp_flight_min)/(l0_virtual - l_min)+((kp_flight_max - kp_flight_min)/(l0_virtual - l_min)*l0_virtual+kp_flight_min)
  F_virtual [N] : Outport
  wires:
  k_virtual3/1 -> Extra Damping At Max Extension/1
  Sum3/1 -> F_virtual [N]/1
  Extra Damping At Max Extension/1 -> Sum3/2
  Constant7/1 -> Extra Damping At Max Extension/3
  Compare To Constant/1 -> Extra Damping At Max Extension/2
  Switch During Escape Phase/1 -> Sum15/1
  Constant5/1 -> MinMax1/2
  MinMax1/1 -> Product1/2
  Constant4/1 -> MinMax/2
  MinMax/1 -> MinMax1/1
  Product1/1 -> Sum2/1
  kp_flight_function/1 -> MinMax/1
  Fcn/1 -> Product/1
  Sum15/1 -> k_virtual/1, Product1/1
  Leg Length [m m/s]/1 -> Demux2/1
  Demux2/1 -> Compare To Constant/1, Fcn/1, Sum15/2, kp_flight_function/1
  Sum1/1 -> Switch For Flight/3
  Constant1/1 -> Sum4/1
  Demux2/2 -> Sum4/2
  k_virtual/1 -> Sum1/1
  Sum4/1 -> k_virtual2/1, Product/2, k_virtual3/1
  k_virtual2/1 -> Sum1/2
  Flight [1/0]/1 -> Switch For Flight/2
  Escape [1/0]/1 -> Switch During Escape Phase/2
  Constant2/1 -> Switch During Escape Phase/3
  Constant3/1 -> Switch During Escape Phase/1
  Product/1 -> Sum2/2
  Switch For Flight/1 -> Sum3/1
  Sum2/1 -> Switch For Flight/1

== system raibert_hopper_2d/Control/Behavior Control/Primary Secondary Leg Swap/Toggle ==
  Trigger : TriggerPort  TriggerType=falling  PortDimensions=1
  Logical Operator : Logic  Operator=NOT  AllPortsSameDT=off  OutDataTypeStr=boolean
  Memory : Memory  X0=1  InheritSampleTime=on
  "[1/0]" : Outport  InitialOutput=[1]
  wires:
  Logical Operator/1 -> "[1/0]"/1, Memory/1
  Memory/1 -> Logical Operator/1

== system raibert_hopper_2d/Control/Behavior Control/Secondary Leg Behavior/Leg Angle PD ==
  Desired Angle : Inport
  Desired Velocity : Inport  Port=2
  Leg Angle [rad rad/s] : Inport  Port=3
  Demux1 : Demux  Outputs=2
  Gain6 : Gain  Gain=kp_leg_angle
  Gain7 : Gain  Gain=kd_leg_angle
  Sum7 : Sum  Inputs=|+-
  Sum8 : Sum  Inputs=|+-
  Sum9 : Sum  Inputs=|++
  Commanded Leg Torque [Nm] : Outport
  wires:
  Gain6/1 -> Sum9/1
  Sum7/1 -> Gain6/1
  Demux1/1 -> Sum7/2
  Sum9/1 -> Commanded Leg Torque [Nm]/1
  Desired Velocity/1 -> Sum8/1
  Sum8/1 -> Gain7/1
  Desired Angle/1 -> Sum7/1
  Gain7/1 -> Sum9/2
  Demux1/2 -> Sum8/2
  Leg Angle [rad rad/s]/1 -> Demux1/1

== system raibert_hopper_2d/Control/Behavior Control/Secondary Leg Behavior/Leg Length PD ==
  Desired Length : Inport
  Desired Velocity : Inport  Port=2
  Leg Length [m m/s] : Inport  Port=3
  Demux1 : Demux  Outputs=2
  Sum7 : Sum  Inputs=|+-
  Sum8 : Sum  Inputs=|+-
  Sum9 : Sum
  kd_leg_length_secondary : Gain  Gain=kd_leg_length_secondary
  kp_leg_length_secondary : Gain  Gain=kp_leg_length_secondary
  Commanded Force [N] : Outport
  wires:
  Leg Length [m m/s]/1 -> Demux1/1
  Demux1/2 -> Sum8/2  "l_dot_measured"
  kd_leg_length_secondary/1 -> Sum9/2
  Desired Length/1 -> Sum7/1
  Sum8/1 -> kd_leg_length_secondary/1
  Desired Velocity/1 -> Sum8/1
  Sum9/1 -> Commanded Force [N]/1
  Demux1/1 -> Sum7/2  "l_measured"
  Sum7/1 -> kp_leg_length_secondary/1
  kp_leg_length_secondary/1 -> Sum9/1

== system raibert_hopper_2d/Control/Behavior Control/Velocity Estimation/Recursive Moving Average ==
  dx [m/s] : Inport
  Delay : Delay  DelayLength=dx_avg_samples  InitialCondition=0  UseCircularBuffer=on  SampleTime=sample_time
  Gain : Gain  Gain=1/dx_avg_samples
  Sum : Sum  Inputs=-++
  Unit Delay : UnitDelay  SampleTime=sample_time
  dx_avg [m/s] : Outport
  wires:
  Unit Delay/1 -> Sum/3
  Gain/1 -> dx_avg [m/s]/1
  Delay/1 -> Sum/1
  Sum/1 -> Unit Delay/1, Gain/1
  dx [m/s]/1 -> Sum/2, Delay/1

== system raibert_hopper_2d/Control/Behavior Control/Primary Leg Behavior/Leg Placement Torque/Leg Angle PD ==
  Desired Angle : Inport
  Desired Velocity : Inport  Port=2
  Leg Angle [rad rad/s] : Inport  Port=3
  Demux1 : Demux  Outputs=2
  Sum7 : Sum  Inputs=|+-
  Sum8 : Sum  Inputs=|+-
  Sum9 : Sum
  kd_leg_angle : Gain  Gain=kd_leg_angle
  kp_leg_angle : Gain  Gain=kp_leg_angle
  Commanded Leg Torque [Nm] : Outport
  wires:
  kp_leg_angle/1 -> Sum9/1
  Sum7/1 -> kp_leg_angle/1
  Demux1/1 -> Sum7/2
  Sum9/1 -> Commanded Leg Torque [Nm]/1
  Desired Velocity/1 -> Sum8/1
  Sum8/1 -> kd_leg_angle/1
  Desired Angle/1 -> Sum7/1
  kd_leg_angle/1 -> Sum9/2
  Demux1/2 -> Sum8/2
  Leg Angle [rad rad/s]/1 -> Demux1/1

== system raibert_hopper_2d/Control/Behavior Control/Primary Leg Behavior/Leg Thrust/Thrust Timer ==
  Enable : EnablePort  StatesWhenEnabling=reset  ShowOutputPort=on
  Constant : Constant
  Discrete-Time Integrator : DiscreteIntegrator  IntegratorMethod=Accumulation: Forward Euler  gainval=sample_time  ExternalReset=rising  SampleTime=sample_time
  timer [s] : Outport  InitialOutput=[0]
  wires:
  Constant/1 -> Discrete-Time Integrator/1
  Enable/1 -> Discrete-Time Integrator/2
  Discrete-Time Integrator/1 -> timer [s]/1

== stateflow chart raibert_hopper_2d/Control/Behavior Control/Primary Leg Behavior/Raibert  Hopper State Machine ==
  state Loading
    entry: placement = false;
    entry: posture = false;
    entry: thrust = false;
    entry: flight = false;
    entry: escape = false;
  state Compression
    entry: placement = false;
    entry: posture = true;
    entry: thrust = false;
    entry: flight = false;
    entry: escape = false;
  state Thrust
    entry: placement = false;
    entry: posture = true;
    entry: thrust = true;
    entry: flight = false;
    entry: escape = false;
  state Unloading
    entry: placement = false;
    entry: posture = false;
    entry: thrust = true;
    entry: flight = false;
    entry: escape = false;
  state Escape
    entry: placement = false;
    entry: posture = false;
    entry: thrust = false;
    entry: flight = true;
    entry: escape = true;
  state Flight
    entry: placement = true;
    entry: posture = false;
    entry: thrust = false;
    entry: flight = true;
    entry: escape = false;
  (junction 91) -> Loading
  Loading -> (junction 130) [order 2] : [Fy < contact_threshold]
  (junction 93) -> (junction 91)
  (junction 130) -> (junction 128)
  Loading -> Compression [order 1] : [Fy > loaded_threshold]
  (junction 115) -> Compression
  (junction 118) -> (junction 115)
  Compression -> Thrust : [dl >= 0 && dl_prev < 0]
  Thrust -> Unloading [order 1] : [Fy < loaded_threshold]
  Thrust -> (junction 102) [order 2] : [l > l_max]
  (junction 102) -> (junction 100)
  (junction 122) -> (junction 118)
  Unloading -> Escape [order 1] : [Fy < contact_threshold || l > l_max]
  Unloading -> (junction 122) [order 2] : [Fy > loaded_threshold && dl < 0]
  Escape -> Flight : after(t_flight,sec)
  (junction 100) -> Escape
  (default) -> Flight
  Flight -> (junction 93) : [Fy > contact_threshold]
  (junction 128) -> Flight
  data: flight output; escape output; thrust output; posture output; l input; dl input; dl_prev input; Fy input; t_flight parameter; placement output boolean; l_max parameter; contact_threshold parameter; loaded_threshold parameter

== matlab function raibert_hopper_2d/Control/Behavior Control/Lateral Control ==
  data: tau_r output size=1; qLateralR input; dqLateralR input; qLateralL input; dqLateralL input; F_leg input; l_leg input; placement input; escape input; right_or_left input; lateral_target_angle_right parameter; lateral_target_angle_left parameter; boom_mount_angle parameter; boom_pelvis_offset_angle parameter; l_yaw_center_to_pelvis parameter; m_leg_motor parameter; g parameter; lateral_offset parameter; tau_l output size=1; kp_lateral parameter; kd_lateral parameter; minimum_lateral_angle parameter; maximum_lateral_angle parameter; HIP_MTR_MAX_CONT_TORQUE parameter
function [tau_r, tau_l] = LateralBoomControl(qLateralR, dqLateralR, qLateralL, dqLateralL, F_leg, l_leg, placement, escape, right_or_left, lateral_target_angle_right, lateral_target_angle_left, boom_mount_angle, boom_pelvis_offset_angle, l_yaw_center_to_pelvis, m_leg_motor, g, lateral_offset, kp_lateral, kd_lateral, minimum_lateral_angle, maximum_lateral_angle, HIP_MTR_MAX_CONT_TORQUE)

    gravity_compensation = m_leg_motor*g*lateral_offset;
    
    % Right placement
    desired = saturate([lateral_target_angle_right, 0],minimum_lateral_angle,maximum_lateral_angle);
    measured = [qLateralR, dqLateralR];
    tau_r = [kp_lateral, kd_lateral] * (desired-measured)' + gravity_compensation;
    tau_r = max(min(HIP_MTR_MAX_CONT_TORQUE, tau_r),-HIP_MTR_MAX_CONT_TORQUE);
    
    % Left placement
    desired = saturate([lateral_target_angle_left, 0],minimum_lateral_angle,maximum_lateral_angle);
    measured = [qLateralL, dqLateralL];
    tau_l = [kp_lateral, kd_lateral] * (desired-measured)' + gravity_compensation;
    tau_l = max(min(HIP_MTR_MAX_CONT_TORQUE, tau_l),-HIP_MTR_MAX_CONT_TORQUE);
    
    % Stance
    if ~escape
        if ~placement && right_or_left
            angle = qLateralR - boom_pelvis_offset_angle + boom_mount_angle;
            J =   (l_leg - l_yaw_center_to_pelvis*sin(angle)) ./ (l_leg.*l_yaw_center_to_pelvis.*cos(angle) - l_yaw_center_to_pelvis*lateral_offset*sin(angle));    
            tau_r = -F_leg*(J - lateral_offset) + gravity_compensation;
        elseif ~placement && ~right_or_left
            angle = qLateralL + boom_pelvis_offset_angle - boom_mount_angle;
            J =  -(l_leg + l_yaw_center_to_pelvis*sin(angle)) ./ (l_leg.*l_yaw_center_to_pelvis.*cos(angle) - l_yaw_center_to_pelvis*lateral_offset*sin(angle));  
            tau_l = F_leg*(J - lateral_offset) + gravity_compensation;
        end
    end
end

function [desired_saturated] = saturate(desired, minimum_lateral_angle, maximum_lateral_angle)
    desired_saturated = desired;
    if desired(1) < minimum_lateral_angle
        desired_saturated = [minimum_lateral_angle, 0];
    elseif desired(1) > maximum_lateral_angle
        desired_saturated = [maximum_lateral_angle, 0];    
    end
end

== matlab function raibert_hopper_2d/Control/Behavior Control/Torque Distribution Right/Motor Torque Saturation Optimization ==
  data: x1s input; t1 output; x2s input; lambda1 parameter; lambda2 parameter; max_torque_sagittal parameter; t2 output
% Optimal leg motor torque distribution
function [t1, t2] = distribute_torque(x1s, x2s, lambda1, lambda2, max_torque_sagittal)

s = max_torque_sagittal;

% possible solutions
x1 = [                                                      x1s;
                                                            0;
                                                            s;
                                                            0;
                                                           -s;
  (lambda2*s + lambda1*x1s - lambda2*x2s)/(lambda1 + lambda2);
  (lambda1*x1s - lambda2*s + lambda2*x2s)/(lambda1 + lambda2);
  (lambda2*s + lambda1*x1s + lambda2*x2s)/(lambda1 + lambda2);
 -(lambda2*s - lambda1*x1s + lambda2*x2s)/(lambda1 + lambda2)];
 
x2 = [                                                      x2s;
                                                            s;
                                                            0;
                                                           -s;
                                                            0;
  (lambda1*s - lambda1*x1s + lambda2*x2s)/(lambda1 + lambda2);
  (lambda1*s + lambda1*x1s + lambda2*x2s)/(lambda1 + lambda2);
  (lambda1*x1s - lambda1*s + lambda2*x2s)/(lambda1 + lambda2);
 -(lambda1*s + lambda1*x1s - lambda2*x2s)/(lambda1 + lambda2)];

% test constraints
c1 = s - x1 - x2 >= 0;
c2 = s + x1 + x2 >= 0;
c3 = s - x1 + x2 >= 0;
c4 = s + x1 - x2 >= 0;
constraints = c1 & c2 & c3 & c4;

% objective function to maximize
f = -lambda1*(x1-x1s).^2-lambda2*(x2-x2s).^2;
satisfied = find(constraints);
[~,I] = max(f(satisfied));

t1 = x1(satisfied(I));
t2 = x2(satisfied(I));

== matlab function raibert_hopper_2d/Control/Behavior Control/Velocity Estimation/dx_from_yaw_and_roll ==
  data: qRoll input; dx output; dqYaw input; dqPitch input; l_boom_projected parameter; d_y_boom_com_offset parameter
function dx = fcn(qRoll, dqYaw, dqPitch, l_boom_projected, d_y_boom_com_offset)
    dx = l_boom_projected*(dqYaw*cos(qRoll)) - dqPitch*d_y_boom_com_offset;
